simulink library "Lib_LPF"  (R2024a)
settings: Solver=VariableStepAuto  StartTime=0.0  StopTime=10.0  RelTol=1e-3
undefined symbols (not defined in the file): C01HVSWF
settings Model: Creator=30610  LastModifiedBy=admin
settings DebuggingCC: UnconnectedInputMsg=warning  UnconnectedOutputMsg=warning  UnconnectedLineMsg=warning
settings ModelReferenceCC: EnableRefExpFcnMdlSchedulingChecks=on
settings RTWCC: GPUComputeCapability=3.5  DLArmComputeVersion=19.05

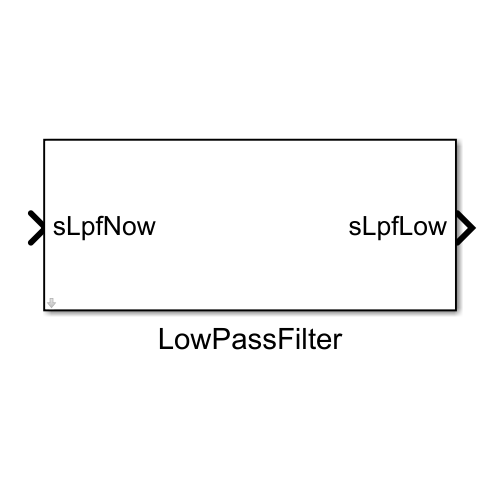
[thumbnail: Simulink's stored preview of the top-level diagram]
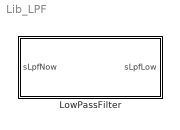
== system Lib_LPF ==
  LowPassFilter : Subsystem  mask{La=C01HVSWF.sHVdcLa, Lb=C01HVSWF.sHVdcLb, Init_Value=C01HVSWF.sVdcInit}
      mask prompts: La "Gain_La"; Lb "Gain_Lb"
      mask DialogControl Container4 Prompt: LPF Discrete-time realization​
      mask DialogControl Control3 Prompt: y(n) = Laㆍy(n-1) + Lbㆍ(x(n)+x(n-1))
      mask DialogControl Control4 Prompt: La = (2-Tsw)/(2+Tsw)
      mask DialogControl Control5 Prompt: Lb = Tsw/(2+Tsw)
      mask DialogControl Container6 Prompt: Low Pass Filter Gain

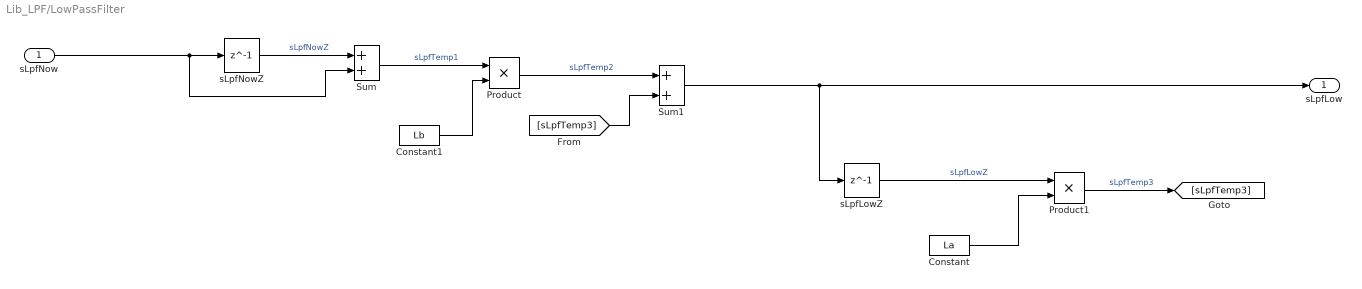
== system Lib_LPF/LowPassFilter ==
  sLpfNow : Inport  OutDataTypeStr=single
  Constant : Constant  Value=La  OutDataTypeStr=single
  Constant1 : Constant  Value=Lb  OutDataTypeStr=single
  Product : Product
  Product1 : Product
  Sum : Sum
  Sum1 : Sum
  sLpfLowZ : Delay  DelayLength=1  InitialCondition=Init_Value  StateName=sLpfLowZ
  sLpfNowZ : Delay  DelayLength=1  InitialCondition=Init_Value  StateName=sLpfNowZ
  sLpfLow : Outport  OutDataTypeStr=single  VectorParamsAs1DForOutWhenUnconnected=off
  wires:
  sLpfLowZ/1 -> Product1/1  "sLpfLowZ"
  Constant/1 -> Product1/2
  Sum1/1 -> sLpfLow/1, sLpfLowZ/1
  Product/1 -> Sum1/1  "sLpfTemp2"
  Constant1/1 -> Product/2
  Sum/1 -> Product/1  "sLpfTemp1"
  sLpfNowZ/1 -> Sum/1  "sLpfNowZ"
  sLpfNow/1 -> sLpfNowZ/1, Sum/2
  Product1/1 -> [sLpfTemp3]  "sLpfTemp3"
  [sLpfTemp3] -> Sum1/2
